simulink model "P3SysID"  (Simulink 8.0)
settings: Solver=VariableStepDiscrete  StartTime=0.0  StopTime=TStop  MaxStep=Ts  RelTol=1e-3
values from neighbouring files (symbols this model uses):
  Ts = 1/100    (= 0.01)    [SysIDP3.m]
libraries: cstblocks x2, slident x1
settings Model: Creator=samnazari  LastModifiedBy=sqn4594
settings OptimizationCC: ExpressionDepthLimit=128
settings CodeAppCC: CustomSymbolStrType=$N$R$M_T

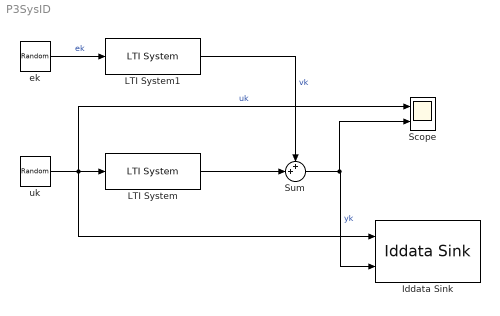
== system P3SysID ==
  Iddata Sink : slident/Iddata Sink  datasetname=P3Data  Ts=Ts  isu=on  isy=on
  LTI System : cstblocks/LTI System  sys=BA  IC=[]
  LTI System1 : cstblocks/LTI System  sys=AC  IC=[]
  Scope : Scope  NumInputPorts=2
      settings: YMin=-5~-5  YMax=5~5  SaveName=y_true
  Sum : Sum  Inputs=++|
  ek : RandomNumber  Variance=0.64  SampleTime=Ts
  uk : RandomNumber  SampleTime=Ts
  wires:
  uk/1 -> Scope/1, Iddata Sink/1, LTI System/1  "uk"
  LTI System/1 -> Sum/2
  LTI System1/1 -> Sum/1  "vk"
  ek/1 -> LTI System1/1  "ek"
  Sum/1 -> Scope/2, Iddata Sink/2  "yk"
